simulink model "gm_sampleModel1777_2_sub"  (R2023a)
settings: Solver=VariableStepAuto  StartTime=0.0  StopTime=10.0  RelTol=1e-3
libraries: simulink x2
settings Model: Creator=user1  LastModifiedBy=user1
settings OptimizationCC: BlockReduction=off  ConditionallyExecuteInputs=off
settings DebuggingCC: InheritedTsInSrcMsg=none

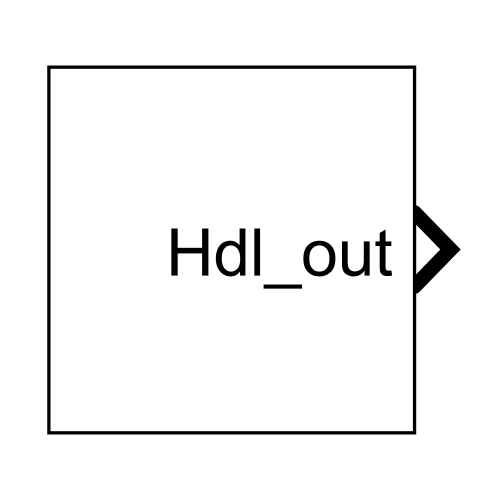
[thumbnail: Simulink's stored preview of the top-level diagram]
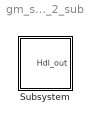
== system gm_sampleModel1777_2_sub ==
  Subsystem : Subsystem

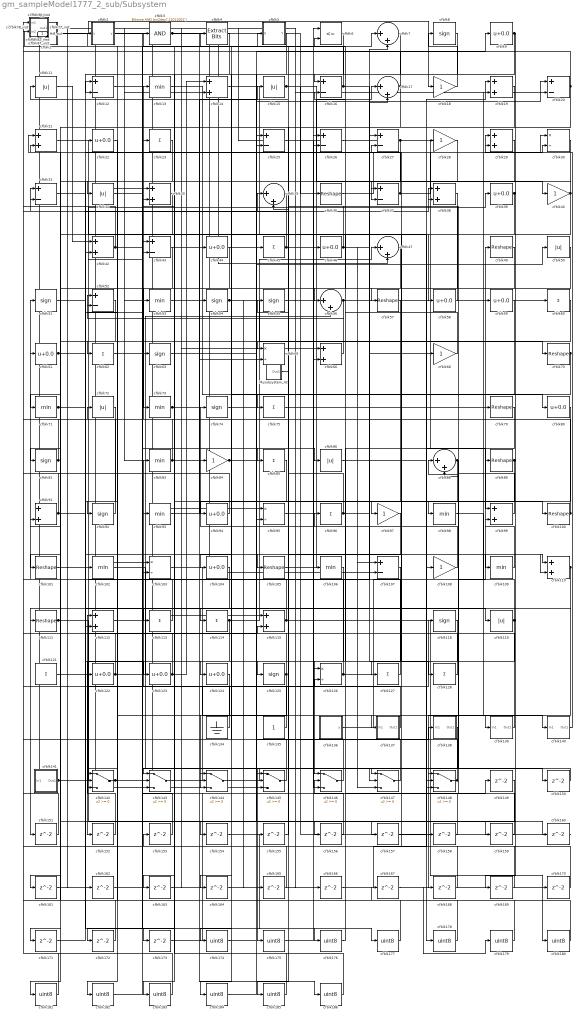
== system gm_sampleModel1777_2_sub/Subsystem ==
  Mysubsystem_42 : Subsystem
  cfblk1 : Subsystem  mask(Detect Rise Nonnegative){vinit=double(0), InputProcessing=Elements as channels (sample based), OutDataTypeStr=uint8}
      mask prompts: vinit "Simulink:masks:InitialCondition_MP"; InputProcessing "Simulink:masks:InputProcessing_MP"; OutDataTypeStr "Simulink:masks:OutputDataType_MP"
      mask help: Simulink:masks:DetectRiseNonnegative_MD
      mask init:
      | InputProcessing = 'Elements as channels (sample based)';
      | OutDataTypeStr = 'uint8';
      | vinit = double(0);
      mask TypeOptions InputProcessing: Simulink:masks:ColumnsAsChannelsFrameBased | Simulink:masks:ElementsAsChannelsSampleBased
      mask TypeOptions OutDataTypeStr: Simulink:masks:uint8 | Simulink:masks:boolean
      mask Display: fprintf('U >= 0\n&  NOT\nU/z >= 0')
  cfblk{36,49,57,70,79,89,100..101,105,111} (10 alike) : Reshape
  cfblk{13,53,71,73,83,93,98,102,106,109} (10 alike) : MinMax  OutDataTypeStr=uint8
  cfblk{30,65,95,103,126} (5 alike) : Product  Inputs=*/  OutDataTypeStr=uint8  RndMeth=Zero  SaturateOnIntegerOverflow=on
  cfblk{9,22,39,44,46,58..59,61,80,94,104,122..124} (14 alike) : Bias  Bias=0.0  SaturateOnIntegerOverflow=off
  cfblk{12,16,20,25..27,31,37,43,52,107} (11 alike) : Sum  Inputs=+-  OutDataTypeStr=uint8
  cfblk{18,28,40,68,84,97,108} (7 alike) : Gain  OutDataTypeStr=uint8
  cfblk10_inst : Subsystem
  cfblk{11,15,32,50,72,86,119} (7 alike) : Abs  OutDataTypeStr=uint8  SaturateOnIntegerOverflow=off
  cfblk{14,19,21,29,33,38,42,66,91,99,110,112,115} (13 alike) : Sum  OutDataTypeStr=uint8
  cfblk{23,45,60,62,75,85,96,113..114,121,127..128} (12 alike) : Sum  Inputs=+  OutDataTypeStr=uint8
  cfblk116_inst : Subsystem
  cfblk117_inst : Subsystem
  cfblk{8,51,54..55,63,74,81,92,118,125} (10 alike) : Signum
  cfblk120_inst : Subsystem
  cfblk134 : Ground
  cfblk135 : Constant  OutDataTypeStr=uint8  SampleTime=-1
  cfblk136 : Subsystem  mask(Counter Limited){uplimit=double(7), tsamp=double(-1)}
      mask prompts: uplimit "Simulink:masks:UpperLimit_MP"; tsamp "Simulink:masks:SampleTime_MP"
      mask help: Simulink:masks:CounterLimited_MD
      mask init:
      | nbits = double(8);
      | tsamp = double(-1);
      | uplimit = double(7);
  cfblk137 : Subsystem
  cfblk138 : Subsystem
  cfblk139 : Subsystem
  cfblk140 : Subsystem
  cfblk141 : Subsystem
  cfblk{142..148} (7 alike) : Switch  OutDataTypeStr=uint8  SaturateOnIntegerOverflow=off  InputSameDT=off
  cfblk{149..173} (25 alike) : Delay  SampleTime=1
  cfblk{7,17,35,47,56,88} (6 alike) : Sum  Inputs=|++  OutDataTypeStr=uint8
  cfblk{174..186} (13 alike) : DataTypeConversion  OutDataTypeStr=uint8  SaturateOnIntegerOverflow=off  RndMeth=Floor
  cfblk2 : Subsystem  mask(Compare To Constant){relop=<=, const=double(3), OutDataTypeStr=uint8, ZeroCross=on}
      mask prompts: relop "Simulink:masks:Operator_MP"; const "Simulink:masks:ConstantValue_MP"; OutDataTypeStr "Simulink:masks:OutputDataType_MP"; ZeroCross "Simulink:masks:EnableZerocrossingDetection_MP"
      mask help: Simulink:masks:CompareToConstant_MD
      mask init:
      | OutDataTypeStr = 'uint8';
      | ZeroCross = 'on';
      | blkName = 'sampleModel1777_2_sub/Subsystem/cfblk2';
      | const = double(3);
      | const_str = '3.0';
      | const_val = double(3);
      | relop = '<=';
      | setValue = 'fixdt(0, 8)';
      | str = '<= 3';
      mask TypeOptions relop: == | ~= | < | <= | >= | >
      mask TypeOptions OutDataTypeStr: Simulink:masks:uint8 | Simulink:masks:boolean
      mask Callback ZeroCross: sl('zeroCrossEnable', gcbh);
      mask Display: disp(str)
  cfblk3 : simulink/Logic and Bit Operations/Bitwise Operator  logicop=AND  UseBitMask=on  BitMask=bin2dec('11011001')  BitMaskRealWorld=Stored Integer
      settings: LibrarySourceBlock=|
      | hdlsllib/Logic and Bit
      | Operations/Bitwise
      | Operator
  cfblk34_inst : Subsystem
  cfblk4 : simulink/Logic and Bit Operations/Extract Bits  bitsToExtract=Upper half  numBits=8  bitIdxRange=[0 7]  outScalingMode=Preserve fixed-point scaling
      settings: LibrarySourceBlock=|
      | hdlsllib/Logic and Bit
      | Operations/Extract Bits
  cfblk41_inst : Subsystem
  cfblk5 : Subsystem  mask(Detect Fall Negative){vinit=double(0), InputProcessing=Elements as channels (sample based), OutDataTypeStr=uint8}
      mask prompts: vinit "Simulink:masks:InitialCondition_MP"; InputProcessing "Simulink:masks:InputProcessing_MP"; OutDataTypeStr "Simulink:masks:OutputDataType_MP"
      mask help: Simulink:masks:DetectFallNegative_MD
      mask init:
      | InputProcessing = 'Elements as channels (sample based)';
      | OutDataTypeStr = 'uint8';
      | vinit = double(0);
      mask TypeOptions InputProcessing: Simulink:masks:ColumnsAsChannelsFrameBased | Simulink:masks:ElementsAsChannelsSampleBased
      mask TypeOptions OutDataTypeStr: Simulink:masks:uint8 | Simulink:masks:boolean
      mask Display: fprintf('U < 0\n&  NOT\nU/z < 0')
  cfblk6 : RelationalOperator  Operator=<=  OutDataTypeStr=boolean  InputSameDT=off
  cfblk64_inst : Subsystem
  cfblk67_inst : Subsystem
  cfblk69_inst : Subsystem
  cfblk76_inst : Subsystem
  cfblk77_inst : Subsystem
  cfblk78_inst : Subsystem
  cfblk82_inst : Subsystem
  cfblk87_inst : Subsystem
  cfblk90_inst : Subsystem
  Hdl_out : Outport  OutDataTypeStr=uint8  SampleTime=1
  wires:
  Mysubsystem_42/1(Out1) -> cfblk76_inst/2(in2)
  cfblk1/1(Y) -> cfblk18/1
  cfblk10_inst/1(out1) -> cfblk41_inst/1(in1), cfblk143/3
  cfblk100/1 -> cfblk51/1, cfblk98/1, cfblk13/1
  cfblk101/1 -> cfblk39/1
  cfblk102/1 -> cfblk172/1
  cfblk103/1 -> cfblk139/1(In1)
  cfblk104/1 -> cfblk151/1
  cfblk105/1 -> cfblk17/1
  cfblk106/1 -> cfblk146/1
  cfblk107/1 -> cfblk152/1
  cfblk108/1 -> cfblk74/1
  cfblk109/1 -> cfblk49/1
  cfblk11/1 -> cfblk42/1
  cfblk110/1 -> cfblk111/1, cfblk169/1, cfblk168/1
  cfblk111/1 -> cfblk43/2, cfblk160/1
  cfblk112/1 -> cfblk175/1
  cfblk113/1 -> cfblk78_inst/2(in2)
  cfblk114/1 -> cfblk47/1, cfblk163/1
  cfblk115/1 -> cfblk33/2, cfblk180/1
  cfblk116_inst/1(out1) -> cfblk115/1
  cfblk117_inst/1(out1) -> cfblk107/2, cfblk102/1, cfblk45/1
  cfblk118/1 -> cfblk185/1
  cfblk119/1 -> cfblk88/1, cfblk124/1
  cfblk12/1 -> cfblk23/1
  cfblk120_inst/1(out1) -> cfblk47/2, cfblk145/3
  cfblk121/1 -> cfblk126/2
  cfblk122/1 -> cfblk67_inst/1(in1), cfblk56/2, cfblk52/1
  cfblk123/1 -> cfblk64_inst/2(in2), cfblk14/1
  cfblk124/1 -> cfblk182/1
  cfblk125/1 -> cfblk77_inst/1(in1), cfblk144/3
  cfblk126/1 -> cfblk99/2, cfblk69_inst/2(in2), cfblk21/2
  cfblk127/1 -> cfblk61/1
  cfblk128/1 -> cfblk10_inst/1(in1)
  cfblk13/1 -> cfblk80/1
  cfblk134/1 -> cfblk87_inst/1(in1)
  cfblk135/1 -> cfblk43/1
  cfblk136/1(y) -> cfblk59/1
  cfblk137/1(Out1) -> cfblk83/1
  cfblk138/1(Out1) -> cfblk183/1
  cfblk139/1(Out1) -> cfblk93/1
  cfblk14/1 -> cfblk178/1
  cfblk140/1(Out1) -> cfblk29/1
  cfblk141/1(Out1) -> cfblk7/2, cfblk115/2
  cfblk142/1 -> cfblk158/1, cfblk157/1
  cfblk143/1 -> cfblk118/1
  cfblk144/1 -> cfblk150/1
  cfblk145/1 -> cfblk64_inst/1(in1)
  cfblk146/1 -> cfblk35/2
  cfblk147/1 -> cfblk4/1
  cfblk148/1 -> cfblk82_inst/2(in2), cfblk96/1
  cfblk149/1 -> cfblk181/1
  cfblk15/1 -> cfblk37/2, cfblk36/1
  cfblk150/1 -> cfblk147/1
  cfblk151/1 -> cfblk78_inst/1(in1)
  cfblk152/1 -> cfblk112/1
  cfblk153/1 -> cfblk143/2
  cfblk154/1 -> cfblk176/1
  cfblk155/1 -> cfblk35/1
  cfblk156/1 -> cfblk146/2
  cfblk157/1 -> cfblk19/1
  cfblk158/1 -> cfblk16/2
  cfblk159/1 -> cfblk88/2
  cfblk16/1 -> cfblk79/1, cfblk69_inst/1(in1)
  cfblk160/1 -> cfblk1/1(U)
  cfblk161/1 -> cfblk42/2
  cfblk162/1 -> cfblk103/2
  cfblk163/1 -> cfblk26/2
  cfblk164/1 -> cfblk25/2
  cfblk165/1 -> cfblk77_inst/2(in2)
  cfblk166/1 -> cfblk148/3
  cfblk167/1 -> cfblk179/1
  cfblk168/1 -> cfblk148/2
  cfblk169/1 -> cfblk27/2
  cfblk17/1 -> cfblk34_inst/1(in1), cfblk65/1
  cfblk170/1 -> cfblk91/2
  cfblk171/1 -> cfblk12/1
  cfblk172/1 -> cfblk31/1
  cfblk173/1 -> cfblk66/2
  cfblk174/1 -> cfblk50/1
  cfblk175/1 -> cfblk6/1
  cfblk176/1 -> cfblk6/2
  cfblk177/1 -> cfblk72/1
  cfblk178/1 -> cfblk2/1(u)
  cfblk179/1 -> cfblk67_inst/2(in2)
  cfblk18/1 -> cfblk8/1
  cfblk180/1 -> cfblk167/1
  cfblk181/1 -> cfblk90_inst/1(in1)
  cfblk182/1 -> cfblk149/1
  cfblk183/1 -> cfblk90_inst/2(in2)
  cfblk184/1 -> cfblk138/1(In1)
  cfblk185/1 -> cfblk3/1
  cfblk186/1 -> cfblk153/1
  cfblk19/1 -> cfblk101/1
  cfblk2/1(y) -> cfblk177/1
  cfblk20/1 -> cfblk82_inst/1(in1), cfblk104/1
  cfblk21/1 -> cfblk108/1
  cfblk22/1 -> cfblk92/1
  cfblk23/1 -> cfblk112/2
  cfblk25/1 -> cfblk46/1
  cfblk26/1 -> cfblk40/1
  cfblk27/1 -> cfblk99/1, cfblk32/1, cfblk75/1
  cfblk28/1 -> cfblk62/1
  cfblk29/1 -> cfblk171/1
  cfblk3/1 -> cfblk186/1, Hdl_out/1
  cfblk30/1 -> cfblk144/2
  cfblk31/1 -> cfblk25/1
  cfblk32/1 -> cfblk147/2
  cfblk33/1 -> cfblk161/1
  cfblk34_inst/1(out1) -> cfblk20/2, cfblk14/2
  cfblk35/1 -> cfblk31/2
  cfblk36/1 -> cfblk30/2
  cfblk37/1 -> cfblk29/2, cfblk21/1
  cfblk38/1 -> cfblk73/1
  cfblk39/1 -> cfblk56/1, cfblk142/3
  cfblk4/1 -> cfblk63/1
  cfblk40/1 -> cfblk58/1, cfblk37/1, cfblk127/1
  cfblk41_inst/1(out1) -> cfblk54/1, cfblk166/1
  cfblk42/1 -> cfblk86/1, cfblk7/1, cfblk10_inst/2(in2)
  cfblk43/1 -> cfblk81/1
  cfblk44/1 -> cfblk113/1
  cfblk45/1 -> cfblk116_inst/1(in1), cfblk109/1
  cfblk46/1 -> cfblk27/1, cfblk147/3, cfblk117_inst/1(in1), cfblk110/1
  cfblk47/1 -> cfblk57/1
  cfblk49/1 -> cfblk94/1
  cfblk5/1(Y) -> cfblk184/1
  cfblk50/1 -> cfblk122/1
  cfblk51/1 -> cfblk38/1
  cfblk52/1 -> cfblk71/1
  cfblk53/1 -> cfblk15/1
  cfblk54/1 -> cfblk70/1, cfblk165/1
  cfblk55/1 -> cfblk106/1
  cfblk56/1 -> cfblk52/2, cfblk107/1, cfblk68/1
  cfblk57/1 -> cfblk144/1
  cfblk58/1 -> cfblk11/1
  cfblk59/1 -> cfblk145/1
  cfblk6/1 -> cfblk174/1
  cfblk60/1 -> cfblk142/1
  cfblk61/1 -> cfblk123/1, cfblk105/1
  cfblk62/1 -> cfblk30/1
  cfblk63/1 -> cfblk20/1
  cfblk64_inst/1(out1) -> cfblk162/1
  cfblk65/1 -> cfblk155/1
  cfblk66/1 -> cfblk5/1(U)
  cfblk67_inst/1(out1) -> cfblk95/1, cfblk103/1
  cfblk68/1 -> cfblk26/1
  cfblk69_inst/1(out1) -> cfblk60/1
  cfblk7/1 -> cfblk145/2
  cfblk70/1 -> cfblk164/1, cfblk114/1
  cfblk71/1 -> cfblk173/1, cfblk53/1
  cfblk72/1 -> cfblk142/2
  cfblk73/1 -> cfblk65/2, cfblk85/1
  cfblk74/1 -> cfblk156/1
  cfblk75/1 -> cfblk19/2
  cfblk76_inst/1(out1) -> cfblk33/1, cfblk22/1, cfblk121/1
  cfblk77_inst/1(out1) -> cfblk84/1, cfblk170/1, cfblk141/1(In1)
  cfblk78_inst/1(out1) -> cfblk66/1
  cfblk79/1 -> cfblk126/1
  cfblk8/1 -> cfblk12/2
  cfblk80/1 -> cfblk97/1
  cfblk81/1 -> cfblk76_inst/1(in1), cfblk41_inst/2(in2), cfblk116_inst/2(in2)
  cfblk82_inst/1(out1) -> cfblk28/1
  cfblk83/1 -> cfblk117_inst/2(in2), cfblk100/1
  cfblk84/1 -> cfblk9/1, cfblk110/2
  cfblk85/1 -> cfblk154/1
  cfblk86/1 -> cfblk89/1
  cfblk87_inst/1(out1) -> cfblk120_inst/1(in1)
  cfblk88/1 -> cfblk148/1, cfblk146/3
  cfblk89/1 -> cfblk143/1, cfblk95/2
  cfblk9/1 -> cfblk16/1, cfblk159/1
  cfblk90_inst/1(out1) -> cfblk91/1
  cfblk91/1 -> cfblk34_inst/2(in2), cfblk119/1
  cfblk92/1 -> cfblk87_inst/2(in2)
  cfblk93/1 -> cfblk44/1
  cfblk94/1 -> cfblk120_inst/2(in2)
  cfblk95/1 -> cfblk137/1(In1)
  cfblk96/1 -> cfblk55/1, cfblk17/2, cfblk128/1
  cfblk97/1 -> cfblk125/1
  cfblk98/1 -> cfblk140/1(In1)
  cfblk99/1 -> cfblk38/2

== system gm_sampleModel1777_2_sub/Subsystem/Mysubsystem_42 ==
  cfblk133 : Constant  Value=0  VectorParams1D=off  OutDataTypeStr=uint8  SampleTime=1
  Out1 : Outport  SampleTime=1
  wires:
  cfblk133/1 -> Out1/1

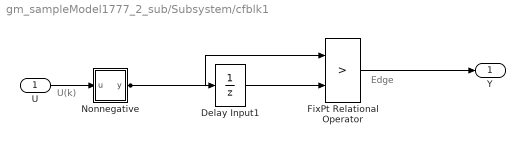
== system gm_sampleModel1777_2_sub/Subsystem/cfblk1 ==
  note: U(k)
  note: Edge
  U : Inport  OutDataTypeStr=uint8  SampleTime=1
  Delay Input1 : UnitDelay  Description=Store in Global RAM  DisableCoverage=on  InitialCondition=vinit  SampleTime=-1  HasFrameUpgradeWarning=on
  FixPt Relational Operator : RelationalOperator  Operator=>  OutDataTypeStr=fixdt(0, 8)  ZeroCross=off  InputSameDT=off
  Nonnegative : Subsystem  mask(Compare To Zero){relop=>=, OutDataTypeStr=boolean, ZeroCross=off}
      mask prompts: relop "Simulink:masks:Operator_MP"; OutDataTypeStr "Simulink:masks:OutputDataType_MP"; ZeroCross "Simulink:masks:EnableZerocrossingDetection_MP"
      mask help: Simulink:masks:CompareToZero_MD
      mask init:
      | OutDataTypeStr = 'boolean';
      | ZeroCross = 'off';
      | blkName = 'sampleModel1777_2_sub/Subsystem/cfblk1/Nonnegative';
      | relop = '>=';
      | setValue = 'boolean';
      mask TypeOptions relop: == | ~= | < | <= | >= | >
      mask TypeOptions OutDataTypeStr: Simulink:masks:uint8 | Simulink:masks:boolean
      mask Callback ZeroCross: sl('zeroCrossEnable', gcbh);
      mask Display: disp([relop,' 0'])
  Y : Outport  SampleTime=1
  wires:
  U/1 -> Nonnegative/1(u)
  Delay Input1/1 -> FixPt Relational Operator/2
  FixPt Relational Operator/1 -> Y/1
  Nonnegative/1(y) -> FixPt Relational Operator/1, Delay Input1/1

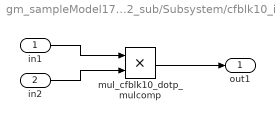
== system gm_sampleModel1777_2_sub/Subsystem/cfblk10_inst ==
  in1 : Inport  OutDataTypeStr=uint8  SampleTime=1
  in2 : Inport  Port=2  OutDataTypeStr=uint8  SampleTime=1
  mul_cfblk10_dotp_mulcomp : Product  Inputs=**  OutDataTypeStr=uint8  SampleTime=1
  out1 : Outport  OutDataTypeStr=uint8  SampleTime=1
  wires:
  in1/1 -> mul_cfblk10_dotp_mulcomp/1
  in2/1 -> mul_cfblk10_dotp_mulcomp/2
  mul_cfblk10_dotp_mulcomp/1 -> out1/1

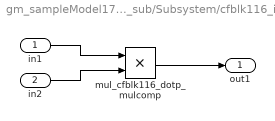
== system gm_sampleModel1777_2_sub/Subsystem/cfblk116_inst ==
  in1 : Inport  OutDataTypeStr=uint8  SampleTime=1
  in2 : Inport  Port=2  OutDataTypeStr=uint8  SampleTime=1
  mul_cfblk116_dotp_mulcomp : Product  Inputs=**  OutDataTypeStr=uint8  SampleTime=1
  out1 : Outport  OutDataTypeStr=uint8  SampleTime=1
  wires:
  in1/1 -> mul_cfblk116_dotp_mulcomp/1
  in2/1 -> mul_cfblk116_dotp_mulcomp/2
  mul_cfblk116_dotp_mulcomp/1 -> out1/1

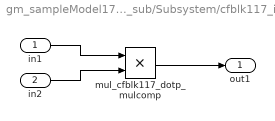
== system gm_sampleModel1777_2_sub/Subsystem/cfblk117_inst ==
  in1 : Inport  OutDataTypeStr=uint8  SampleTime=1
  in2 : Inport  Port=2  OutDataTypeStr=uint8  SampleTime=1
  mul_cfblk117_dotp_mulcomp : Product  Inputs=**  OutDataTypeStr=uint8  SampleTime=1
  out1 : Outport  OutDataTypeStr=uint8  SampleTime=1
  wires:
  in1/1 -> mul_cfblk117_dotp_mulcomp/1
  in2/1 -> mul_cfblk117_dotp_mulcomp/2
  mul_cfblk117_dotp_mulcomp/1 -> out1/1

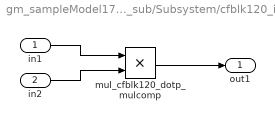
== system gm_sampleModel1777_2_sub/Subsystem/cfblk120_inst ==
  in1 : Inport  OutDataTypeStr=uint8  SampleTime=1
  in2 : Inport  Port=2  OutDataTypeStr=uint8  SampleTime=1
  mul_cfblk120_dotp_mulcomp : Product  Inputs=**  OutDataTypeStr=uint8  SampleTime=1
  out1 : Outport  OutDataTypeStr=uint8  SampleTime=1
  wires:
  in1/1 -> mul_cfblk120_dotp_mulcomp/1
  in2/1 -> mul_cfblk120_dotp_mulcomp/2
  mul_cfblk120_dotp_mulcomp/1 -> out1/1

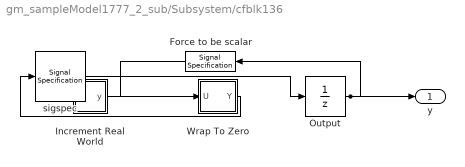
== system gm_sampleModel1777_2_sub/Subsystem/cfblk136 ==
  Force to be scalar : SignalSpecification  DisableCoverage=on  Dimensions=1
  Increment Real World : Subsystem  mask(Real World Value Increment){}
      mask help: Simulink:masks:RealWorldValueIncrement_MD
      mask Display: disp('V++')
  Output : UnitDelay  InitialCondition=0.0  SampleTime=tsamp  HasFrameUpgradeWarning=on
  Wrap To Zero : Subsystem  mask(Wrap To Zero){Threshold=double(7)}
      mask prompts: Threshold "Simulink:masks:Threshold_MP"
      mask help: Simulink:masks:WrapToZero_MD
  sigspec : SignalSpecification  OutDataTypeStr=uint8  Dimensions=1
  y : Outport  SampleTime=1
  wires:
  Force to be scalar/1 -> Increment Real World/1(u)
  Increment Real World/1(y) -> Wrap To Zero/1(U)
  Output/1 -> Force to be scalar/1, y/1
  Wrap To Zero/1(Y) -> sigspec/1
  sigspec/1 -> Output/1

== system gm_sampleModel1777_2_sub/Subsystem/cfblk137 ==
  In1 : Inport  OutDataTypeStr=uint8  PortDimensions=1  SampleTime=1
  Out1 : Outport  SampleTime=1
  wires:
  In1/1 -> Out1/1

== system gm_sampleModel1777_2_sub/Subsystem/cfblk138 ==
  In1 : Inport  OutDataTypeStr=uint8  PortDimensions=1  SampleTime=1
  Out1 : Outport  SampleTime=1
  wires:
  In1/1 -> Out1/1

== system gm_sampleModel1777_2_sub/Subsystem/cfblk139 ==
  In1 : Inport  OutDataTypeStr=uint8  PortDimensions=1  SampleTime=1
  Out1 : Outport  SampleTime=1
  wires:
  In1/1 -> Out1/1

== system gm_sampleModel1777_2_sub/Subsystem/cfblk140 ==
  In1 : Inport  OutDataTypeStr=uint8  PortDimensions=1  SampleTime=1
  Out1 : Outport  SampleTime=1
  wires:
  In1/1 -> Out1/1

== system gm_sampleModel1777_2_sub/Subsystem/cfblk141 ==
  In1 : Inport  OutDataTypeStr=uint8  PortDimensions=1  SampleTime=1
  Out1 : Outport  SampleTime=1
  wires:
  In1/1 -> Out1/1

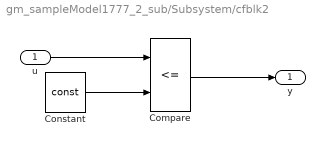
== system gm_sampleModel1777_2_sub/Subsystem/cfblk2 ==
  u : Inport  OutDataTypeStr=uint8  SampleTime=1
  Compare : RelationalOperator  Operator=<=  OutDataTypeStr=fixdt(0, 8)
  Constant : Constant  DisableCoverage=on  Value=const  OutDataTypeStr=Inherit: Inherit via back propagation  SampleTime=-1
  y : Outport  SampleTime=1
  wires:
  u/1 -> Compare/1
  Compare/1 -> y/1
  Constant/1 -> Compare/2

== system gm_sampleModel1777_2_sub/Subsystem/cfblk34_inst ==
  in1 : Inport  OutDataTypeStr=uint8  SampleTime=1
  in2 : Inport  Port=2  OutDataTypeStr=uint8  SampleTime=1
  mul_cfblk34_dotp_mulcomp : Product  Inputs=**  OutDataTypeStr=uint8  SampleTime=1
  out1 : Outport  OutDataTypeStr=uint8  SampleTime=1
  wires:
  in1/1 -> mul_cfblk34_dotp_mulcomp/1
  in2/1 -> mul_cfblk34_dotp_mulcomp/2
  mul_cfblk34_dotp_mulcomp/1 -> out1/1

== system gm_sampleModel1777_2_sub/Subsystem/cfblk41_inst ==
  in1 : Inport  OutDataTypeStr=uint8  SampleTime=1
  in2 : Inport  Port=2  OutDataTypeStr=uint8  SampleTime=1
  mul_cfblk41_dotp_mulcomp : Product  Inputs=**  OutDataTypeStr=uint8  SampleTime=1
  out1 : Outport  OutDataTypeStr=uint8  SampleTime=1
  wires:
  in1/1 -> mul_cfblk41_dotp_mulcomp/1
  in2/1 -> mul_cfblk41_dotp_mulcomp/2
  mul_cfblk41_dotp_mulcomp/1 -> out1/1

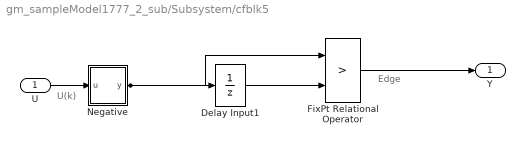
== system gm_sampleModel1777_2_sub/Subsystem/cfblk5 ==
  note: U(k)
  note: Edge
  U : Inport  OutDataTypeStr=uint8  SampleTime=1
  Delay Input1 : UnitDelay  Description=Store in Global RAM  DisableCoverage=on  InitialCondition=vinit  SampleTime=-1  HasFrameUpgradeWarning=on
  FixPt Relational Operator : RelationalOperator  Operator=>  OutDataTypeStr=fixdt(0, 8)  ZeroCross=off  InputSameDT=off
  Negative : Subsystem  mask(Compare To Zero){relop=<, OutDataTypeStr=boolean, ZeroCross=off}
      mask prompts: relop "Simulink:masks:Operator_MP"; OutDataTypeStr "Simulink:masks:OutputDataType_MP"; ZeroCross "Simulink:masks:EnableZerocrossingDetection_MP"
      mask help: Simulink:masks:CompareToZero_MD
      mask init:
      | OutDataTypeStr = 'boolean';
      | ZeroCross = 'off';
      | blkName = 'sampleModel1777_2_sub/Subsystem/cfblk5/Negative';
      | relop = '<';
      | setValue = 'boolean';
      mask TypeOptions relop: == | ~= | < | <= | >= | >
      mask TypeOptions OutDataTypeStr: Simulink:masks:uint8 | Simulink:masks:boolean
      mask Callback ZeroCross: sl('zeroCrossEnable', gcbh);
      mask Display: disp([relop,' 0'])
  Y : Outport  SampleTime=1
  wires:
  U/1 -> Negative/1(u)
  Delay Input1/1 -> FixPt Relational Operator/2
  FixPt Relational Operator/1 -> Y/1
  Negative/1(y) -> FixPt Relational Operator/1, Delay Input1/1

== system gm_sampleModel1777_2_sub/Subsystem/cfblk64_inst ==
  in1 : Inport  OutDataTypeStr=uint8  SampleTime=1
  in2 : Inport  Port=2  OutDataTypeStr=uint8  SampleTime=1
  mul_cfblk64_dotp_mulcomp : Product  Inputs=**  OutDataTypeStr=uint8  SampleTime=1
  out1 : Outport  OutDataTypeStr=uint8  SampleTime=1
  wires:
  in1/1 -> mul_cfblk64_dotp_mulcomp/1
  in2/1 -> mul_cfblk64_dotp_mulcomp/2
  mul_cfblk64_dotp_mulcomp/1 -> out1/1

== system gm_sampleModel1777_2_sub/Subsystem/cfblk67_inst ==
  in1 : Inport  OutDataTypeStr=uint8  SampleTime=1
  in2 : Inport  Port=2  OutDataTypeStr=uint8  SampleTime=1
  mul_cfblk67_dotp_mulcomp : Product  Inputs=**  OutDataTypeStr=uint8  SampleTime=1
  out1 : Outport  OutDataTypeStr=uint8  SampleTime=1
  wires:
  in1/1 -> mul_cfblk67_dotp_mulcomp/1
  in2/1 -> mul_cfblk67_dotp_mulcomp/2
  mul_cfblk67_dotp_mulcomp/1 -> out1/1

== system gm_sampleModel1777_2_sub/Subsystem/cfblk69_inst ==
  in1 : Inport  OutDataTypeStr=uint8  SampleTime=1
  in2 : Inport  Port=2  OutDataTypeStr=uint8  SampleTime=1
  mul_cfblk69_dotp_mulcomp : Product  Inputs=**  OutDataTypeStr=uint8  SampleTime=1
  out1 : Outport  OutDataTypeStr=uint8  SampleTime=1
  wires:
  in1/1 -> mul_cfblk69_dotp_mulcomp/1
  in2/1 -> mul_cfblk69_dotp_mulcomp/2
  mul_cfblk69_dotp_mulcomp/1 -> out1/1

== system gm_sampleModel1777_2_sub/Subsystem/cfblk76_inst ==
  in1 : Inport  OutDataTypeStr=uint8  SampleTime=1
  in2 : Inport  Port=2  OutDataTypeStr=uint8  SampleTime=1
  mul_cfblk76_dotp_mulcomp : Product  Inputs=**  OutDataTypeStr=uint8  SampleTime=1
  out1 : Outport  OutDataTypeStr=uint8  SampleTime=1
  wires:
  in1/1 -> mul_cfblk76_dotp_mulcomp/1
  in2/1 -> mul_cfblk76_dotp_mulcomp/2
  mul_cfblk76_dotp_mulcomp/1 -> out1/1

== system gm_sampleModel1777_2_sub/Subsystem/cfblk77_inst ==
  in1 : Inport  OutDataTypeStr=uint8  SampleTime=1
  in2 : Inport  Port=2  OutDataTypeStr=uint8  SampleTime=1
  mul_cfblk77_dotp_mulcomp : Product  Inputs=**  OutDataTypeStr=uint8  SampleTime=1
  out1 : Outport  OutDataTypeStr=uint8  SampleTime=1
  wires:
  in1/1 -> mul_cfblk77_dotp_mulcomp/1
  in2/1 -> mul_cfblk77_dotp_mulcomp/2
  mul_cfblk77_dotp_mulcomp/1 -> out1/1

== system gm_sampleModel1777_2_sub/Subsystem/cfblk78_inst ==
  in1 : Inport  OutDataTypeStr=uint8  SampleTime=1
  in2 : Inport  Port=2  OutDataTypeStr=uint8  SampleTime=1
  mul_cfblk78_dotp_mulcomp : Product  Inputs=**  OutDataTypeStr=uint8  SampleTime=1
  out1 : Outport  OutDataTypeStr=uint8  SampleTime=1
  wires:
  in1/1 -> mul_cfblk78_dotp_mulcomp/1
  in2/1 -> mul_cfblk78_dotp_mulcomp/2
  mul_cfblk78_dotp_mulcomp/1 -> out1/1

== system gm_sampleModel1777_2_sub/Subsystem/cfblk82_inst ==
  in1 : Inport  OutDataTypeStr=uint8  SampleTime=1
  in2 : Inport  Port=2  OutDataTypeStr=uint8  SampleTime=1
  mul_cfblk82_dotp_mulcomp : Product  Inputs=**  OutDataTypeStr=uint8  SampleTime=1
  out1 : Outport  OutDataTypeStr=uint8  SampleTime=1
  wires:
  in1/1 -> mul_cfblk82_dotp_mulcomp/1
  in2/1 -> mul_cfblk82_dotp_mulcomp/2
  mul_cfblk82_dotp_mulcomp/1 -> out1/1

== system gm_sampleModel1777_2_sub/Subsystem/cfblk87_inst ==
  in1 : Inport  OutDataTypeStr=uint8  SampleTime=1
  in2 : Inport  Port=2  OutDataTypeStr=uint8  SampleTime=1
  mul_cfblk87_dotp_mulcomp : Product  Inputs=**  OutDataTypeStr=uint8  SampleTime=1
  out1 : Outport  OutDataTypeStr=uint8  SampleTime=1
  wires:
  in1/1 -> mul_cfblk87_dotp_mulcomp/1
  in2/1 -> mul_cfblk87_dotp_mulcomp/2
  mul_cfblk87_dotp_mulcomp/1 -> out1/1

== system gm_sampleModel1777_2_sub/Subsystem/cfblk90_inst ==
  in1 : Inport  OutDataTypeStr=uint8  SampleTime=1
  in2 : Inport  Port=2  OutDataTypeStr=uint8  SampleTime=1
  mul_cfblk90_dotp_mulcomp : Product  Inputs=**  OutDataTypeStr=uint8  SampleTime=1
  out1 : Outport  OutDataTypeStr=uint8  SampleTime=1
  wires:
  in1/1 -> mul_cfblk90_dotp_mulcomp/1
  in2/1 -> mul_cfblk90_dotp_mulcomp/2
  mul_cfblk90_dotp_mulcomp/1 -> out1/1

== system gm_sampleModel1777_2_sub/Subsystem/cfblk1/Nonnegative ==
  u : Inport  OutDataTypeStr=uint8  SampleTime=1
  Compare : RelationalOperator  OutDataTypeStr=boolean  ZeroCross=off
  Constant : Constant  DisableCoverage=on  Value=0  OutDataTypeStr=Inherit: Inherit via back propagation  SampleTime=-1  PreserveConstantTs=on
  y : Outport  SampleTime=1
  wires:
  u/1 -> Compare/1
  Compare/1 -> y/1
  Constant/1 -> Compare/2

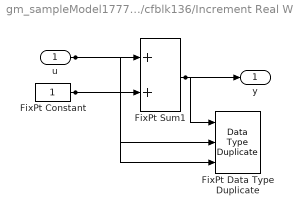
== system gm_sampleModel1777_2_sub/Subsystem/cfblk136/Increment Real World ==
  u : Inport  OutDataTypeStr=uint8  SampleTime=1
  FixPt Constant : Constant  DisableCoverage=on  OutDataTypeStr=Inherit: Inherit via back propagation  SampleTime=-1
  FixPt Data Type Duplicate : DataTypeDuplicate  DisableCoverage=on  NumInputPorts=3
  FixPt Sum1 : Sum  InputSameDT=on  OutDataTypeStr=Inherit: Inherit via back propagation  LockScale=on
  y : Outport  SampleTime=1
  wires:
  u/1 -> FixPt Sum1/1, FixPt Data Type Duplicate/2
  FixPt Constant/1 -> FixPt Sum1/2, FixPt Data Type Duplicate/3
  FixPt Sum1/1 -> FixPt Data Type Duplicate/1, y/1

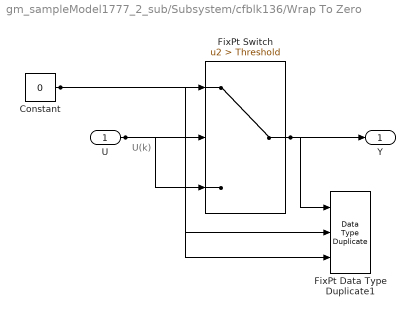
== system gm_sampleModel1777_2_sub/Subsystem/cfblk136/Wrap To Zero ==
  note: U(k)
  U : Inport  OutDataTypeStr=uint8  SampleTime=1
  Constant : Constant  DisableCoverage=on  Value=0  OutDataTypeStr=Inherit: Inherit via back propagation  SampleTime=-1
  FixPt Data Type Duplicate1 : DataTypeDuplicate  DisableCoverage=on  NumInputPorts=3
  FixPt Switch : Switch  Criteria=u2 > Threshold  Threshold=Threshold  OutDataTypeStr=Inherit: Inherit via back propagation  ZeroCross=off  SaturateOnIntegerOverflow=off  InputSameDT=off
  Y : Outport  SampleTime=1
  wires:
  U/1 -> FixPt Switch/3, FixPt Switch/2, FixPt Data Type Duplicate1/2
  Constant/1 -> FixPt Switch/1, FixPt Data Type Duplicate1/3
  FixPt Switch/1 -> FixPt Data Type Duplicate1/1, Y/1

== system gm_sampleModel1777_2_sub/Subsystem/cfblk5/Negative ==
  u : Inport  OutDataTypeStr=uint8  SampleTime=1
  Compare : RelationalOperator  Operator=<  OutDataTypeStr=boolean  ZeroCross=off
  Constant : Constant  DisableCoverage=on  Value=0  OutDataTypeStr=Inherit: Inherit via back propagation  SampleTime=-1  PreserveConstantTs=on
  y : Outport  SampleTime=1
  wires:
  u/1 -> Compare/1
  Compare/1 -> y/1
  Constant/1 -> Compare/2
